simulink model "Accel_model"  (R2016a)
settings: Solver=ode45  StartTime=0.0  StopTime=7  MaxStep=0.01  RelTol=1e-3
values from neighbouring files (symbols this model uses):
  b = e*0.5    (= 0.7925)    [Comparatif.m]    (also in Initialisation_variables_workspace.m = 0.8)
  C_mot = [0,45.126,51.01200000000001,52.974000000000004,51.01200000000001,48.069,49.050000000000004,51.01200000000001,56.898,58.86,58.86,57.879000000000005,56.898,54.936,51.993,48.069,44.145,40.221,36.297000000000004,32.373]    [Initialisation_variables_workspace.m]
  charge_max = 1500    [Comparatif.m]    (also in Initialisation_variables_workspace.m)
  charge_min = 500    [Comparatif.m]    (also in Initialisation_variables_workspace.m = 450)
  ChargePneu = FzMu(1,:)    [Initialisation_variables_workspace.m]
  Cl = 0    [Initialisation_variables_workspace.m]
  coeff_roul = 0.01    [Initialisation_variables_workspace.m]
  Cx = 0.7    [Initialisation_variables_workspace.m]
  g = 9.81    [Initialisation_variables_workspace.m]
  h = (mpilote*h_p)/m    (= 0.3)    [Initialisation_variables_workspace.m]
  J_eq = J_trans + 4*J_rot    (= 4.6575)    [Initialisation_variables_workspace.m]
  m = mtot    (= 60)    [Initialisation_variables_workspace.m]
  maileron = 0    [Initialisation_variables_workspace.m]
  MuLong = FzMu(2,:)    [Initialisation_variables_workspace.m]
  position_initale = 0    [Initialisation_variables_workspace.m]
  R = D_roue/2    (= 0.265)    [Initialisation_variables_workspace.m]
  rap_couronne = 13/45    (= 0.288888888889)    [Initialisation_variables_workspace.m]
  rap_pri = 36/76    (= 0.473684210526)    [Initialisation_variables_workspace.m]
  rapport = [1, 2, 3, 4, 5, 6]    [Initialisation_variables_workspace.m]
  rapport_max = 3    [Initialisation_variables_workspace.m]
  reg_patinage = 8000    [Initialisation_variables_workspace.m]
  reg_rupteur = 14000    [Initialisation_variables_workspace.m]
  regime = [0, 4500:500:13500]    [Initialisation_variables_workspace.m]
  rho = 1.2    [Initialisation_variables_workspace.m]
  S = 0.9    [Initialisation_variables_workspace.m]
  Sproj = 1.8    [Initialisation_variables_workspace.m]
  t_passage = 0.1    [Initialisation_variables_workspace.m]
  v = 1.195    [Comparatif.m]    (also in Initialisation_variables_workspace.m = 1.2)
  v_passage = [0, v1, v2, v3, v4, v5]/3.6    [Initialisation_variables_workspace.m]
  vitesse_initiale = 0    [Initialisation_variables_workspace.m]
undefined symbols (not defined in the file or in its folder): rap
settings Model: Creator=Aurélien  LastModifiedBy=Aurélien

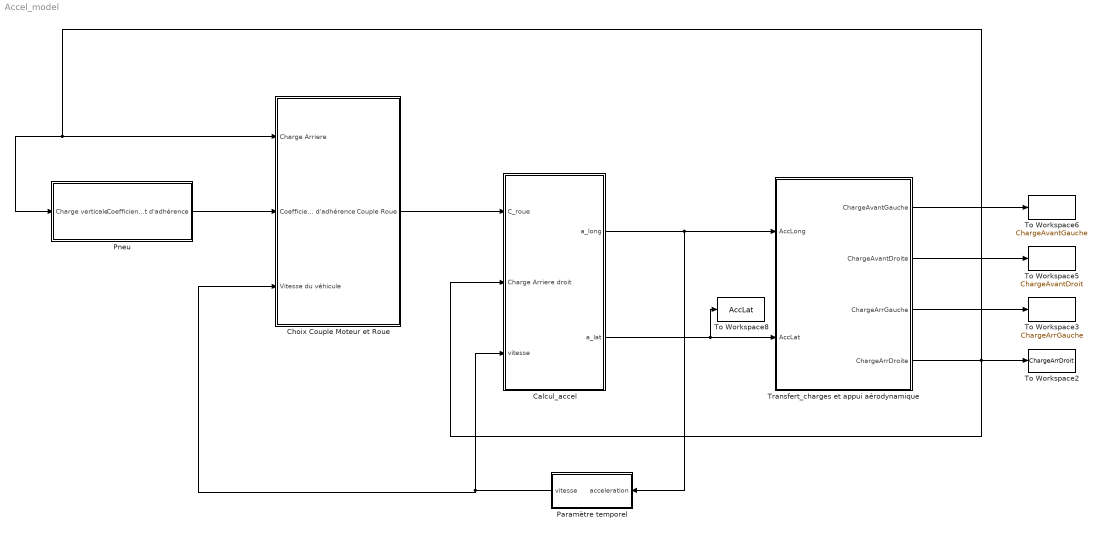
== system Accel_model ==
  Calcul_accel : Subsystem
  "Choix Couple Moteur et Roue " : Subsystem
  "Paramètre temporel " : Subsystem
  Pneu : Subsystem
  To Workspace2 : ToWorkspace  VariableName=ChargeArrDroit  SaveFormat=Timeseries  SampleTime=-1
  To Workspace3 : ToWorkspace  VariableName=ChargeArrGauche  SaveFormat=Timeseries  SampleTime=-1
  To Workspace5 : ToWorkspace  VariableName=ChargeAvantDroit  SaveFormat=Timeseries  SampleTime=-1
  To Workspace6 : ToWorkspace  VariableName=ChargeAvantGauche  SaveFormat=Timeseries  SampleTime=-1
  To Workspace8 : ToWorkspace  VariableName=AccLat  SaveFormat=Timeseries  SampleTime=-1
  Transfert_charges et appui aérodynamique : Subsystem
  wires:
  Transfert_charges et appui aérodynamique/3(ChargeArrGauche) -> To Workspace3/1
  Transfert_charges et appui aérodynamique/2(ChargeAvantDroite) -> To Workspace5/1
  Transfert_charges et appui aérodynamique/1(ChargeAvantGauche) -> To Workspace6/1
  Calcul_accel/2(a_lat) -> To Workspace8/1, Transfert_charges et appui aérodynamique/2(AccLat)
  "Choix Couple Moteur et Roue "/1(Couple Roue) -> Calcul_accel/1(C_roue)
  Pneu/1(Coefficient d'adhérence) -> "Choix Couple Moteur et Roue "/2("Coefficient d'adhérence ")
  "Paramètre temporel "/1("vitesse ") -> "Choix Couple Moteur et Roue "/3(Vitesse du véhicule), Calcul_accel/3(vitesse)
  Calcul_accel/1(a_long) -> Transfert_charges et appui aérodynamique/1(AccLong), "Paramètre temporel "/1(acceleration)
  Transfert_charges et appui aérodynamique/4(ChargeArrDroite) -> Pneu/1(Charge verticale), "Choix Couple Moteur et Roue "/1(Charge Arriere), Calcul_accel/2("Charge Arriere droit "), To Workspace2/1

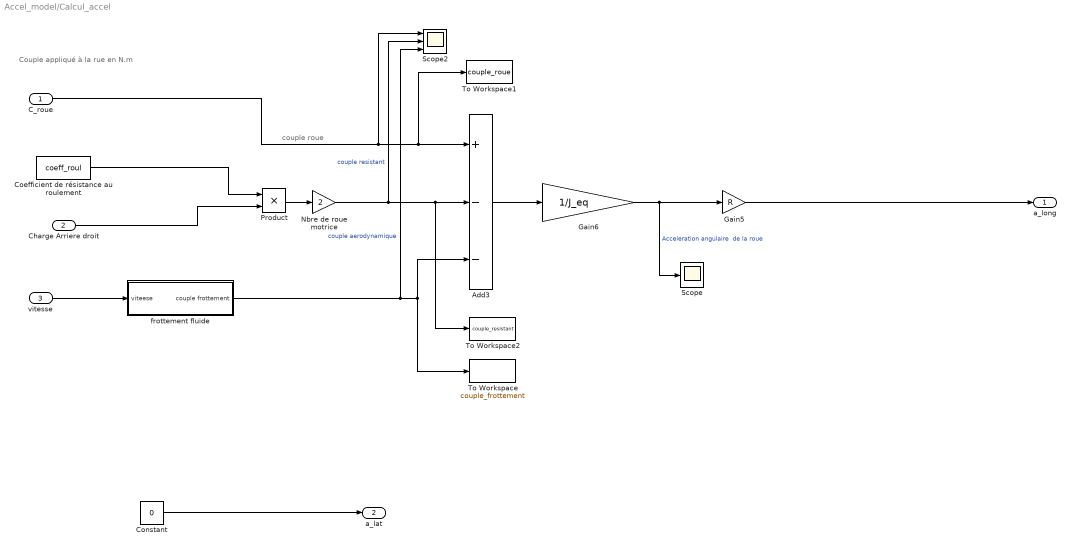
== system Accel_model/Calcul_accel ==
  note: couple roue
  note: Couple appliqué à la rue en N.m
  C_roue : Inport
  "Charge Arriere droit " : Inport  Port=2
  vitesse : Inport  Port=3
  Add3 : Sum  Inputs=+--
  Coefficient de résistance au roulement : Constant  Value=coeff_roul
  Constant : Constant  Value=0
  Gain5 : Gain  Gain=R
  Gain6 : Gain  Gain=1/J_eq
  Nbre de roue motrice : Gain  Gain=2
  Product : Product  Inputs=**
  Scope : Scope
  Scope2 : Scope  NumInputPorts=3
  To Workspace : ToWorkspace  VariableName=couple_frottement  SaveFormat=Timeseries  SampleTime=-1
  To Workspace1 : ToWorkspace  VariableName=couple_roue  SaveFormat=Timeseries  SampleTime=-1
  To Workspace2 : ToWorkspace  VariableName=couple_resistant  SaveFormat=Timeseries  SampleTime=-1
  frottement fluide : Subsystem
  a_long : Outport
  a_lat : Outport  Port=2
  wires:
  Constant/1 -> a_lat/1
  Gain6/1 -> Scope/1, Gain5/1  "Acceleration angulaire  de la roue"
  vitesse/1 -> frottement fluide/1(viteese)
  Coefficient de résistance au roulement/1 -> Product/1
  "Charge Arriere droit "/1 -> Product/2
  Product/1 -> Nbre de roue motrice/1
  C_roue/1 -> Scope2/1, To Workspace1/1, Add3/1
  Nbre de roue motrice/1 -> Scope2/2, To Workspace2/1, Add3/2  "couple resistant"
  Add3/1 -> Gain6/1
  frottement fluide/1(couple frottement) -> Scope2/3, Add3/3, To Workspace/1  "couple aerodynamique"
  Gain5/1 -> a_long/1

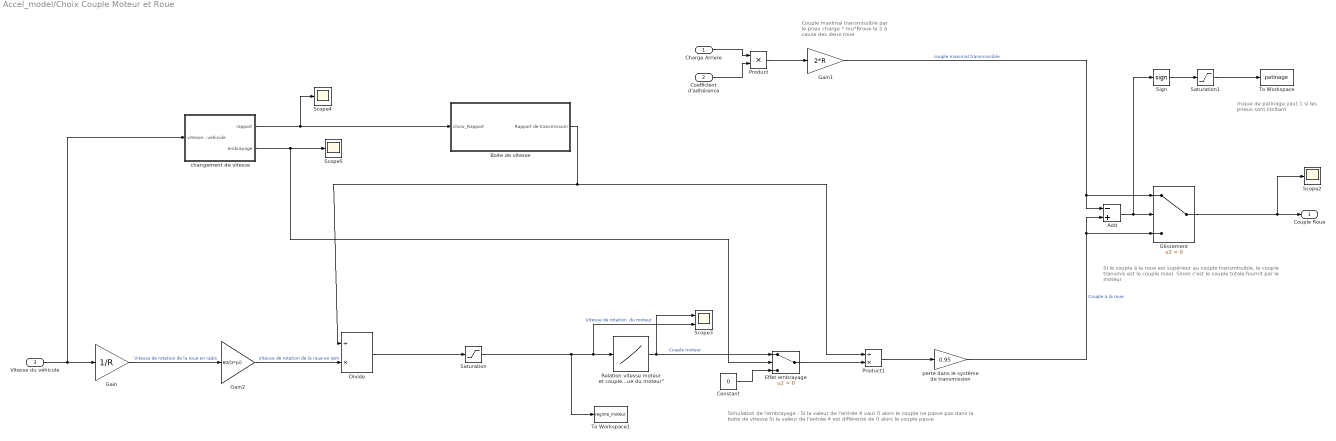
== system Accel_model/Choix Couple Moteur et Roue  ==
  note: risque de patinage
      | vaut 1 si les pneus sont limitant
  note: Simulation de l'embrayage :
      | Si la valeur de l'entrée 4 vaut 0 alors le couple ne passe pas dans la boite de vitesse
      | Si la valeur de l'entrée 4 est différente de 0 alors le couple passe
  note: SI le couple à la roue est supérieur
      | au couple transmissible, le couple transmis est le couple maxi.
      | Sinon c'est le couple totale fournit par le moteur
  note: Couple maximal transmissible
      | par le pneu charge * mu*Rroue
      | le 2 à cause des deux roue
  Charge Arriere : Inport
  "Coefficient d'adhérence " : Inport  Port=2
  Vitesse du véhicule : Inport  Port=3
  Add : Sum  Inputs=-+
  Boite de vitesse : Subsystem
  Constant : Constant  Value=0
  Divide : Product  Inputs=/*
  Effet embrayage : Switch  Criteria=u2 > Threshold
  Gain : Gain  Gain=1/R
  Gain1 : Gain  Gain=2*R
  Gain2 : Gain  Gain=60/(2*pi)
  Glissement : Switch  Criteria=u2 > Threshold
  Product : Product
  Product1 : Product  Inputs=/*
  "Relation vitesse moteur et couple moteur \"Caractéristique du moteur\"" : Lookup_n-D  NumberOfTableDimensions=1  BreakpointsForDimension1=regime  Table=C_mot  InternalRulePriority=Speed  RndMeth=Simplest  InputSameDT=on
  Saturation : Saturate  UpperLimit=reg_rupteur  LowerLimit=reg_patinage
  Saturation1 : Saturate  UpperLimit=1  LowerLimit=0
  Scope2 : Scope
  Scope3 : Scope  NumInputPorts=2
  Scope4 : Scope
  Scope5 : Scope
  Sign : Signum
  To Workspace : ToWorkspace  VariableName=patinage  SaveFormat=Timeseries  SampleTime=-1
  To Workspace1 : ToWorkspace  VariableName=regime_moteur  SaveFormat=Timeseries  SampleTime=-1
  "changement de vitesse " : Subsystem
  perte dans le système de transmission : Gain  Gain=0.95
  Couple Roue : Outport
  wires:
  Add/1 -> Sign/1, Glissement/2
  "changement de vitesse "/1(rapport) -> Scope4/1, Boite de vitesse/1(choix_Rapport)
  Charge Arriere/1 -> Product/1
  "Coefficient d'adhérence "/1 -> Product/2
  Vitesse du véhicule/1 -> Gain/1, "changement de vitesse "/1("vitesse_vehicule ")
  Product/1 -> Gain1/1
  Gain1/1 -> Add/1, Glissement/1  "couple maximal transmissible"
  Boite de vitesse/1(Rapport de transmission) -> Divide/1, Product1/1
  Product1/1 -> perte dans le système de transmission/1
  Glissement/1 -> Scope2/1, Couple Roue/1
  Gain/1 -> Gain2/1  "Vitesse de rotation de la roue en rad/s"
  Divide/1 -> Saturation/1
  Saturation/1 -> To Workspace1/1, Scope3/2, "Relation vitesse moteur et couple moteur \"Caractéristique du moteur\""/1  "Vitesse de rotation  du moteur"
  "Relation vitesse moteur et couple moteur \"Caractéristique du moteur\""/1 -> Effet embrayage/1, Scope3/1  "Couple moteur"
  Effet embrayage/1 -> Product1/2
  "changement de vitesse "/2("embrayage ") -> Effet embrayage/2, Scope5/1
  Gain2/1 -> Divide/2  "Vitesse de rotation de la roue en rpm"
  Constant/1 -> Effet embrayage/3
  Saturation1/1 -> To Workspace/1
  Sign/1 -> Saturation1/1
  perte dans le système de transmission/1 -> Add/2, Glissement/3  "Couple à la roue"

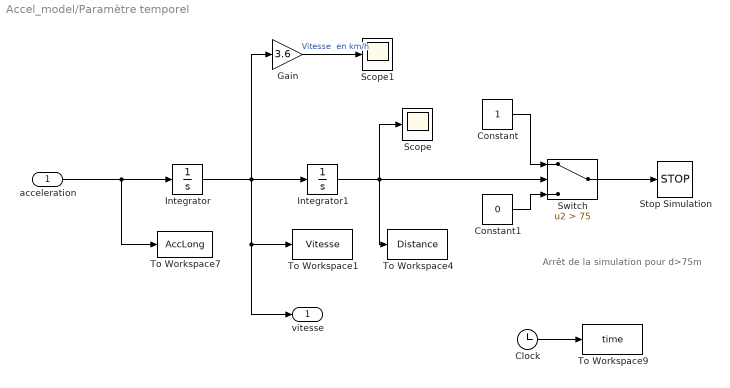
== system Accel_model/Paramètre temporel  ==
  note: Arrêt de la simulation pour d>75m
  acceleration : Inport
  Clock : Clock
  Constant : Constant
  Constant1 : Constant  Value=0
  Gain : Gain  Gain=3.6
  Integrator : Integrator  InitialCondition=vitesse_initiale
  Integrator1 : Integrator  InitialCondition=position_initale
  Scope : Scope
  Scope1 : Scope
  Stop Simulation : Stop
  Switch : Switch  Criteria=u2 > Threshold  Threshold=75
  To Workspace1 : ToWorkspace  VariableName=Vitesse  SaveFormat=Timeseries  SampleTime=-1
  To Workspace4 : ToWorkspace  VariableName=Distance  SaveFormat=Timeseries  SampleTime=-1
  To Workspace7 : ToWorkspace  VariableName=AccLong  SaveFormat=Timeseries  SampleTime=-1
  To Workspace9 : ToWorkspace  VariableName=time  SampleTime=-1
  "vitesse " : Outport
  wires:
  Integrator1/1 -> Scope/1, To Workspace4/1, Switch/2
  Constant/1 -> Switch/1
  acceleration/1 -> Integrator/1, To Workspace7/1
  Integrator/1 -> Gain/1, To Workspace1/1, "vitesse "/1, Integrator1/1
  Constant1/1 -> Switch/3
  Switch/1 -> Stop Simulation/1
  Gain/1 -> Scope1/1  "Vitesse  en km/h"
  Clock/1 -> To Workspace9/1

== system Accel_model/Pneu ==
  Charge verticale : Inport
  1-D Lookup Table : Lookup_n-D  NumberOfTableDimensions=1  BreakpointsForDimension1=ChargePneu  Table=MuLong  InternalRulePriority=Speed  RndMeth=Simplest  InputSameDT=on
  Saturation : Saturate  UpperLimit=charge_max  LowerLimit=charge_min
  Scope4 : Scope
  différence entre tapis de test et piste : Gain  Gain=0.66
  Coefficient d'adhérence : Outport
  wires:
  Saturation/1 -> 1-D Lookup Table/1
  Charge verticale/1 -> Saturation/1
  1-D Lookup Table/1 -> Scope4/1, différence entre tapis de test et piste/1
  différence entre tapis de test et piste/1 -> Coefficient d'adhérence/1

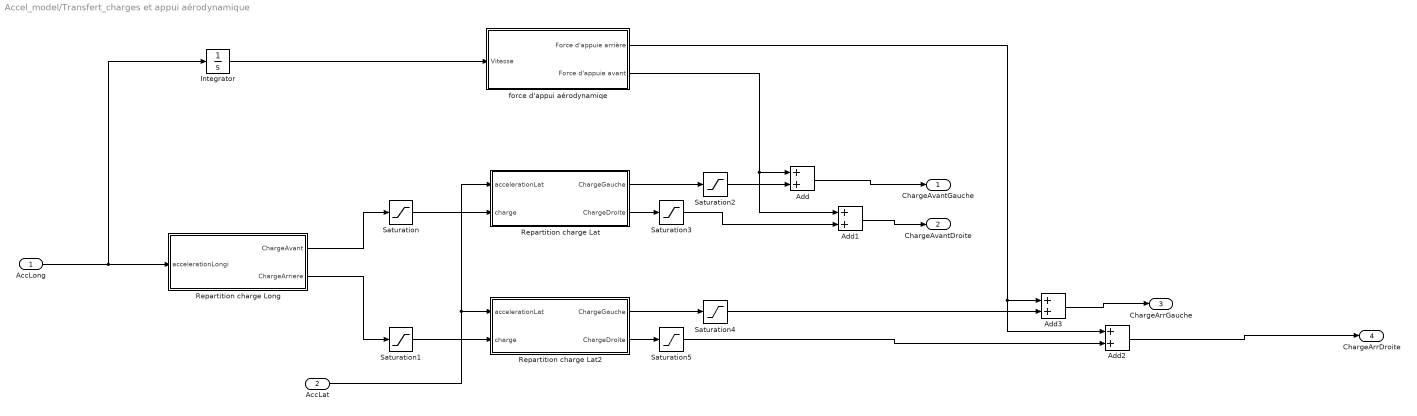
== system Accel_model/Transfert_charges et appui aérodynamique ==
  AccLong : Inport
  AccLat : Inport  Port=2
  Add{,1..3} (4 alike) : Sum
  Integrator : Integrator  InitialCondition=vitesse_initiale
  Repartition charge Lat : Subsystem
  Repartition charge Lat2 : Subsystem
  Repartition charge Long : Subsystem
  Saturation : Saturate  UpperLimit=inf  LowerLimit=0
  Saturation{1..5} (5 alike) : Saturate  UpperLimit=m*g  LowerLimit=0
  force d'appui aérodynamiqe : Subsystem
  ChargeAvantGauche : Outport
  ChargeAvantDroite : Outport  Port=2
  ChargeArrGauche : Outport  Port=3
  ChargeArrDroite : Outport  Port=4
  wires:
  Repartition charge Long/1(ChargeAvant) -> Saturation/1
  Repartition charge Long/2(ChargeArriere) -> Saturation1/1
  AccLong/1 -> Integrator/1, Repartition charge Long/1(accelerationLongi)
  AccLat/1 -> Repartition charge Lat/1(accelerationLat), Repartition charge Lat2/1(accelerationLat)
  Repartition charge Lat/2(ChargeDroite) -> Saturation3/1
  Repartition charge Lat/1(ChargeGauche) -> Saturation2/1
  Repartition charge Lat2/1(ChargeGauche) -> Saturation4/1
  Repartition charge Lat2/2(ChargeDroite) -> Saturation5/1
  Saturation/1 -> Repartition charge Lat/2("charge ")
  Saturation1/1 -> Repartition charge Lat2/2("charge ")
  Integrator/1 -> force d'appui aérodynamiqe/1(Vitesse)
  Saturation2/1 -> Add/2
  force d'appui aérodynamiqe/2(Force d'appuie avant) -> Add/1, Add1/1
  Saturation3/1 -> Add1/2
  Add1/1 -> ChargeAvantDroite/1
  Add/1 -> ChargeAvantGauche/1
  Saturation4/1 -> Add3/2
  force d'appui aérodynamiqe/1(Force d'appuie arrière) -> Add2/1, Add3/1
  Add3/1 -> ChargeArrGauche/1
  Saturation5/1 -> Add2/2
  Add2/1 -> ChargeArrDroite/1

== system Accel_model/Calcul_accel/frottement fluide ==
  viteese : Inport
  Gain : Gain  Gain=(1/2)*rho*Cx*S*R
  Product : Product
  couple frottement : Outport
  wires:
  viteese/1 -> Product/2, Product/1
  Gain/1 -> couple frottement/1
  Product/1 -> Gain/1

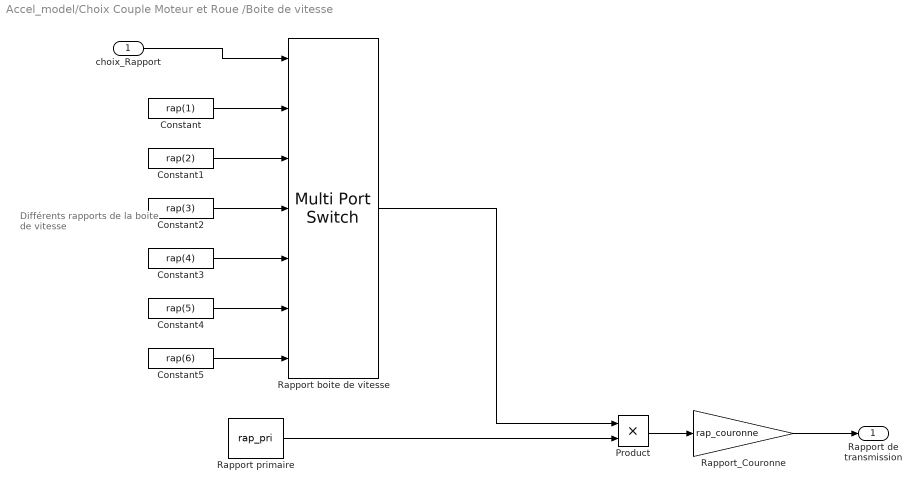
== system Accel_model/Choix Couple Moteur et Roue /Boite de vitesse ==
  note: Différents rapports
      | de la boite de vitesse
  choix_Rapport : Inport
  Constant : Constant  Value=rap(1)
  Constant1 : Constant  Value=rap(2)
  Constant2 : Constant  Value=rap(3)
  Constant3 : Constant  Value=rap(4)
  Constant4 : Constant  Value=rap(5)
  Constant5 : Constant  Value=rap(6)
  Product : Product
  Rapport primaire : Constant  Value=rap_pri
  Rapport boite de vitesse : MultiPortSwitch  Inputs=6
  Rapport_Couronne : Gain  Gain=rap_couronne
  Rapport de transmission : Outport
  wires:
  Constant/1 -> Rapport boite de vitesse/2
  Constant1/1 -> Rapport boite de vitesse/3
  Constant2/1 -> Rapport boite de vitesse/4
  Constant3/1 -> Rapport boite de vitesse/5
  Constant4/1 -> Rapport boite de vitesse/6
  choix_Rapport/1 -> Rapport boite de vitesse/1
  Rapport boite de vitesse/1 -> Product/1
  Rapport_Couronne/1 -> Rapport de transmission/1
  Product/1 -> Rapport_Couronne/1
  Rapport primaire/1 -> Product/2
  Constant5/1 -> Rapport boite de vitesse/7

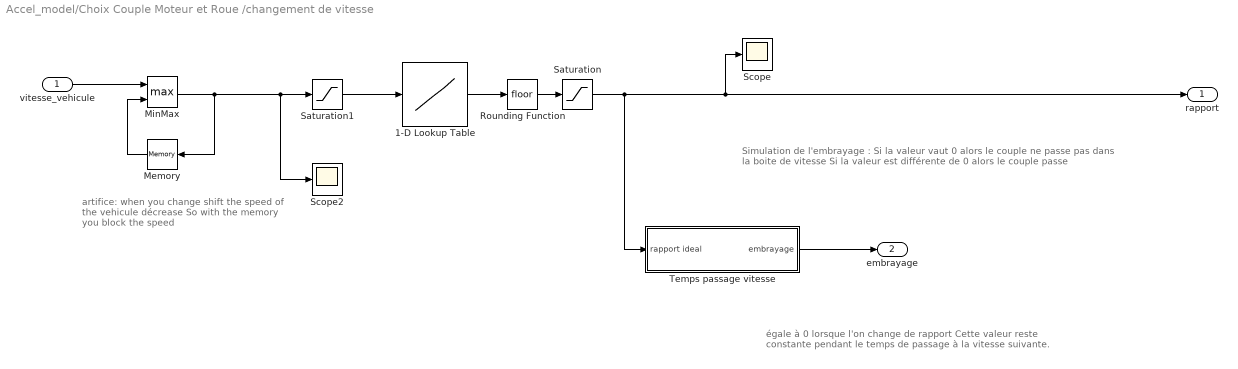
== system Accel_model/Choix Couple Moteur et Roue /changement de vitesse  ==
  note: artifice: when you change shift
      | the speed of the vehicule décrease
      | So with the memory you block the speed
  note: égale à 0 lorsque l'on change de rapport
      | Cette valeur reste constante pendant le temps de passage
      | à la vitesse suivante.
  note: Simulation de l'embrayage :
      | Si la valeur  vaut 0 alors le couple ne passe pas dans la boite de vitesse
      | Si la valeur est différente de 0 alors le couple passe
  "vitesse_vehicule " : Inport
  1-D Lookup Table : Lookup_n-D  NumberOfTableDimensions=1  BreakpointsForDimension1=v_passage  Table=rapport  InternalRulePriority=Speed  RndMeth=Simplest  InputSameDT=on
  Memory : Memory
  MinMax : MinMax  Function=max  Inputs=2
  Rounding Function : Rounding
  Saturation : Saturate  UpperLimit=rapport_max  LowerLimit=1
  Saturation1 : Saturate  UpperLimit=inf  LowerLimit=0
  Scope : Scope
  Scope2 : Scope
  "Temps passage vitesse " : Subsystem
  rapport : Outport
  "embrayage " : Outport  Port=2
  wires:
  "vitesse_vehicule "/1 -> MinMax/1
  1-D Lookup Table/1 -> Rounding Function/1
  Rounding Function/1 -> Saturation/1
  Saturation/1 -> "Temps passage vitesse "/1(rapport ideal), Scope/1, rapport/1
  "Temps passage vitesse "/1(embrayage) -> "embrayage "/1
  Saturation1/1 -> 1-D Lookup Table/1
  MinMax/1 -> Memory/1, Saturation1/1, Scope2/1
  Memory/1 -> MinMax/2

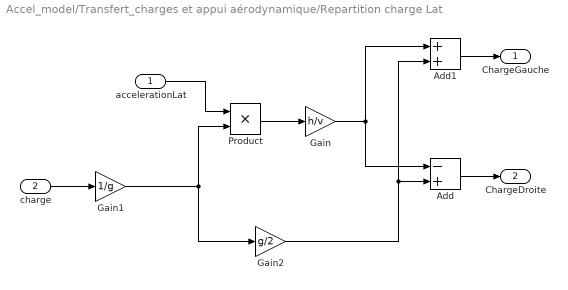
== system Accel_model/Transfert_charges et appui aérodynamique/Repartition charge Lat ==
  accelerationLat : Inport
  "charge " : Inport  Port=2
  Add : Sum  Inputs=-+
  Add1 : Sum
  Gain : Gain  Gain=h/v
  Gain1 : Gain  Gain=1/g
  Gain2 : Gain  Gain=g/2
  Product : Product
  ChargeGauche : Outport
  ChargeDroite : Outport  Port=2
  wires:
  Gain/1 -> Add1/1, Add/1
  Add1/1 -> ChargeGauche/1
  Add/1 -> ChargeDroite/1
  accelerationLat/1 -> Product/1
  "charge "/1 -> Gain1/1
  Product/1 -> Gain/1
  Gain2/1 -> Add1/2, Add/2
  Gain1/1 -> Gain2/1, Product/2

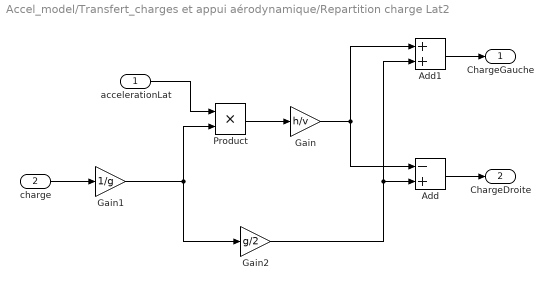
== system Accel_model/Transfert_charges et appui aérodynamique/Repartition charge Lat2 ==
  accelerationLat : Inport
  "charge " : Inport  Port=2
  Add : Sum  Inputs=-+
  Add1 : Sum
  Gain : Gain  Gain=h/v
  Gain1 : Gain  Gain=1/g
  Gain2 : Gain  Gain=g/2
  Product : Product
  ChargeGauche : Outport
  ChargeDroite : Outport  Port=2
  wires:
  Gain/1 -> Add1/1, Add/1
  Add1/1 -> ChargeGauche/1
  Add/1 -> ChargeDroite/1
  accelerationLat/1 -> Product/1
  "charge "/1 -> Gain1/1
  Product/1 -> Gain/1
  Gain2/1 -> Add1/2, Add/2
  Gain1/1 -> Product/2, Gain2/1

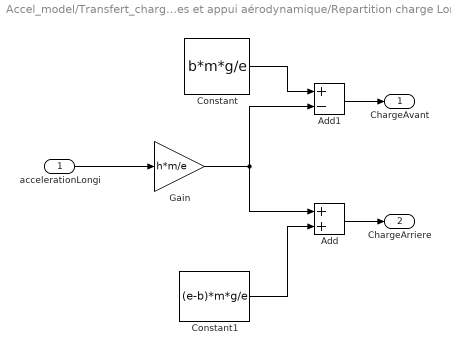
== system Accel_model/Transfert_charges et appui aérodynamique/Repartition charge Long ==
  accelerationLongi : Inport
  Add : Sum
  Add1 : Sum  Inputs=+-
  Constant : Constant  Value=b*m*g/e
  Constant1 : Constant  Value=(e-b)*m*g/e
  Gain : Gain  Gain=h*m/e
  ChargeAvant : Outport
  ChargeArriere : Outport  Port=2
  wires:
  accelerationLongi/1 -> Gain/1
  Gain/1 -> Add/1, Add1/2
  Constant/1 -> Add1/1
  Constant1/1 -> Add/2
  Add1/1 -> ChargeAvant/1
  Add/1 -> ChargeArriere/1

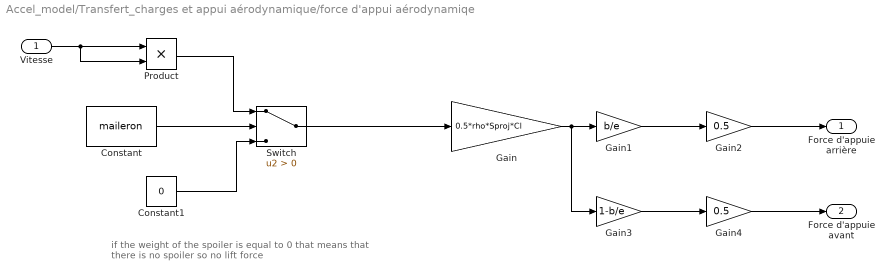
== system Accel_model/Transfert_charges et appui aérodynamique/force d'appui aérodynamiqe ==
  note: if the weight of the spoiler is equal to 0
      | that means that there is no spoiler so no lift force
  Vitesse : Inport
  Constant : Constant  Value=maileron
  Constant1 : Constant  Value=0
  Gain : Gain  Gain=0.5*rho*Sproj*Cl
  Gain1 : Gain  Gain=b/e
  Gain2 : Gain  Gain=0.5
  Gain3 : Gain  Gain=1-b/e
  Gain4 : Gain  Gain=0.5
  Product : Product
  Switch : Switch  Criteria=u2 > Threshold
  Force d'appuie arrière : Outport
  Force d'appuie avant : Outport  Port=2
  wires:
  Vitesse/1 -> Product/1, Product/2
  Gain1/1 -> Gain2/1
  Gain2/1 -> Force d'appuie arrière/1
  Gain/1 -> Gain3/1, Gain1/1
  Gain3/1 -> Gain4/1
  Gain4/1 -> Force d'appuie avant/1
  Switch/1 -> Gain/1
  Product/1 -> Switch/1
  Constant/1 -> Switch/2
  Constant1/1 -> Switch/3

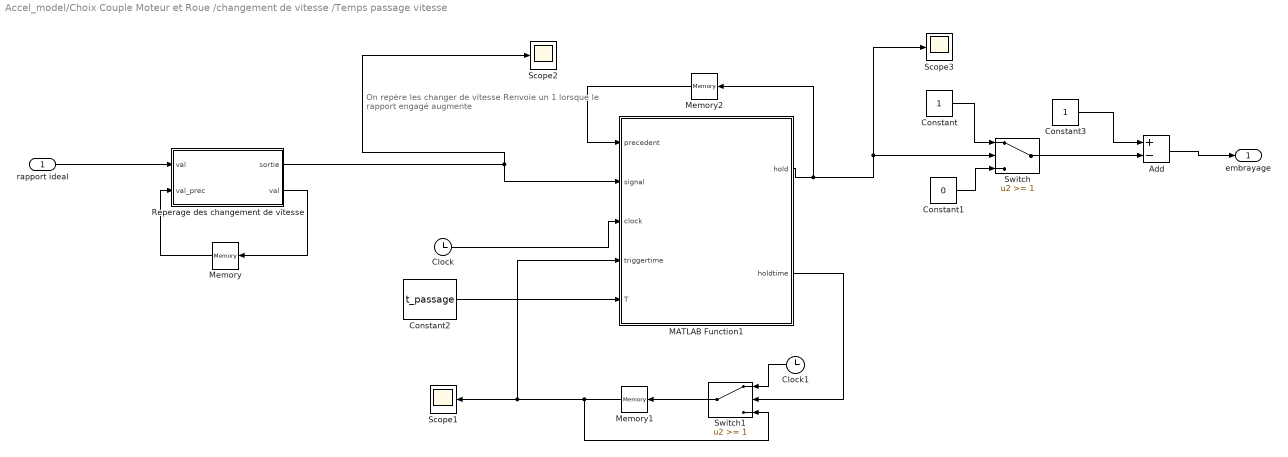
== system Accel_model/Choix Couple Moteur et Roue /changement de vitesse /Temps passage vitesse  ==
  note: On repère les changer de vitesse
      | Renvoie un 1 lorsque le rapport engagé augmente
  rapport ideal : Inport
  Add : Sum  Inputs=+-
  Clock : Clock
  Clock1 : Clock
  Constant : Constant
  Constant1 : Constant  Value=0
  Constant2 : Constant  Value=t_passage
  Constant3 : Constant
  MATLAB Function1 : MATLAB Function  TreatAsAtomicUnit=on
  Memory : Memory  X0=1
  Memory1 : Memory
  Memory2 : Memory
  Reperage des changement de vitesse : MATLAB Function  TreatAsAtomicUnit=on
  Scope1 : Scope
  Scope2 : Scope
  Scope3 : Scope
  Switch : Switch  Threshold=1
  Switch1 : Switch  Threshold=1
  embrayage : Outport
  wires:
  rapport ideal/1 -> Reperage des changement de vitesse/1("val ")
  Memory/1 -> Reperage des changement de vitesse/2(val_prec)
  Reperage des changement de vitesse/2(val) -> Memory/1
  Reperage des changement de vitesse/1(sortie) -> Scope2/1, MATLAB Function1/2(signal)
  MATLAB Function1/1(hold) -> Scope3/1, Switch/2, Memory2/1
  Switch1/1 -> Memory1/1
  MATLAB Function1/2(holdtime) -> Switch1/2
  Constant/1 -> Switch/1
  Constant1/1 -> Switch/3
  Memory1/1 -> Switch1/3, MATLAB Function1/4(triggertime), Scope1/1
  Memory2/1 -> MATLAB Function1/1(precedent)
  Clock1/1 -> Switch1/1
  Clock/1 -> MATLAB Function1/3(clock)
  Constant2/1 -> MATLAB Function1/5(T)
  Switch/1 -> Add/2
  Add/1 -> embrayage/1
  Constant3/1 -> Add/1

== matlab function Accel_model/Choix Couple Moteur et Roue /changement de vitesse /Temps passage vitesse /MATLAB Function1 ==
  data: precedent input; hold output; holdtime output; signal input; clock input; triggertime input; T input
function [hold, holdtime]= fcn(precedent, signal, clock, triggertime, T)
%#Si on repère un changement de rapport, alors on crée un signal créneau ayant la valeur 1 pendant une durée de t_passage

hold = 0;
holdtime = 0;


if signal == 1
    hold = 1;
    holdtime = 1;
end

if precedent == 1 && clock < triggertime + T
    hold = 1;
    holdtime = 0;
end
end

== matlab function Accel_model/Choix Couple Moteur et Roue /changement de vitesse /Temps passage vitesse /Reperage des changement de vitesse ==
  data: val input; sortie output; val_prec input; val output
function [sortie, val]= fcn(val, val_prec)
%#Cette fonction renvoie 1 lorsque l'on change de vitesse
if val == val_prec
    sortie = 0;
else
    sortie = 1;
end
